simulink model "emABS_SB"  (R2023b)
settings: Solver=FixedStepAuto  StartTime=0.0  StopTime=20  FixedStep=0.001  RelTol=1e-3
libraries: Solver_SF x1
settings Model: Creator=황수빈  LastModifiedBy=황수빈

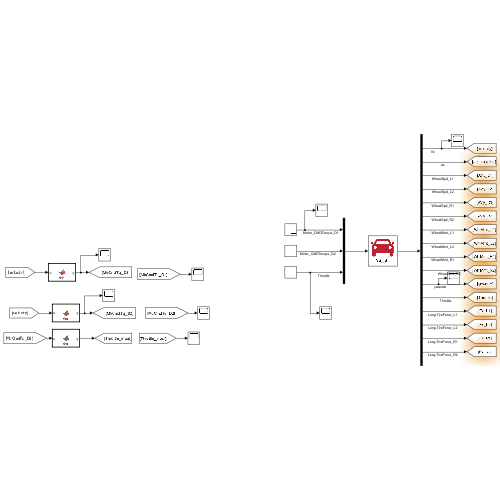
[thumbnail: Simulink's stored preview of the top-level diagram]
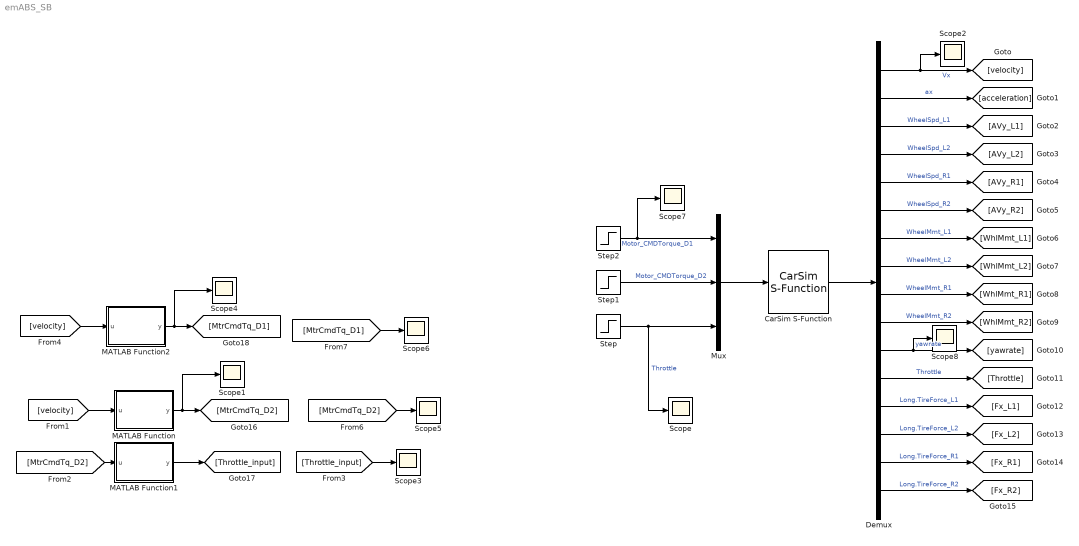
== system emABS_SB ==
  CarSim S-Function : Solver_SF/CarSim S-Function  Priority=1  SIMFILE=simfile.sim  Run_RTs=off  vs_state_ind=Run  StopMode_ind=Vehicle Model
  Demux : Demux  Outputs=16
  MATLAB Function : MATLAB Function  TreatAsAtomicUnit=on
  MATLAB Function1 : MATLAB Function  TreatAsAtomicUnit=on
  MATLAB Function2 : MATLAB Function  TreatAsAtomicUnit=on
  Mux : Mux  Inputs=3
  Scope{,1..8} (9 alike) : Scope
  Step : Step  Time=5  Before=0.8  After=0  SampleTime=0
  Step1 : Step  Time=5  After=-300  SampleTime=5
  Step2 : Step  Time=5  After=-150  SampleTime=5
  wires:
  Mux/1 -> CarSim S-Function/1
  Step1/1 -> Mux/2  "Motor_CMDTorque_D2"
  CarSim S-Function/1 -> Demux/1
  Step/1 -> Scope/1, Mux/3  "Throttle"
  Step2/1 -> Scope7/1, Mux/1  "Motor_CMDTorque_D1"
  Demux/1 -> [velocity], Scope2/1  "Vx"
  Demux/2 -> [acceleration]  "ax"
  Demux/3 -> [AVy_L1]  "WheelSpd_L1"
  Demux/4 -> [AVy_L2]  "WheelSpd_L2"
  Demux/5 -> [AVy_R1]  "WheelSpd_R1"
  Demux/6 -> [AVy_R2]  "WheelSpd_R2"
  Demux/7 -> [WhlMmt_L1]  "WheelMmt_L1"
  Demux/8 -> [WhlMmt_L2]  "WheelMmt_L2"
  Demux/9 -> [WhlMmt_R1]  "WheelMmt_R1"
  Demux/10 -> [WhlMmt_R2]  "WheelMmt_R2"
  Demux/11 -> [yawrate], Scope8/1  "yawrate"
  Demux/12 -> [Throttle]  "Throttle"
  Demux/13 -> [Fx_L1]  "Long.TireForce_L1"
  Demux/14 -> [Fx_L2]  "Long.TireForce_L2"
  Demux/15 -> [Fx_R1]  "Long.TireForce_R1"
  Demux/16 -> [Fx_R2]  "Long.TireForce_R2"
  [velocity] -> MATLAB Function/1(u)
  MATLAB Function/1(y) -> Scope1/1, [MtrCmdTq_D2]
  [MtrCmdTq_D2] -> MATLAB Function1/1(u)
  MATLAB Function1/1(y) -> [Throttle_input]
  [Throttle_input] -> Scope3/1
  [velocity] -> MATLAB Function2/1(u)
  MATLAB Function2/1(y) -> [MtrCmdTq_D1], Scope4/1
  [MtrCmdTq_D2] -> Scope5/1
  [MtrCmdTq_D1] -> Scope6/1

== matlab function emABS_SB/MATLAB Function ==
  data: u input; y output
function y = fcn(u)
if u >=120
    y=-180.5;
else 
    y=0;
end

== matlab function emABS_SB/MATLAB Function2 ==
  data: u input; y output
function y = fcn(u)
if u >=120
    y=-180.5;
else 
    y=0;
end

== matlab function emABS_SB/MATLAB Function1 ==
  data: u input; y output
function y = fcn(u)
if u ~= 0
    y=0;
else
    y=1;
end
